simulink model "sinc3_zdomain"  (R2026a)
settings: Solver=FixedStepDiscrete  StopTime=0.5  FixedStep=5e-07
settings Model: Creator=jinwe  LastModifiedBy=jinwe

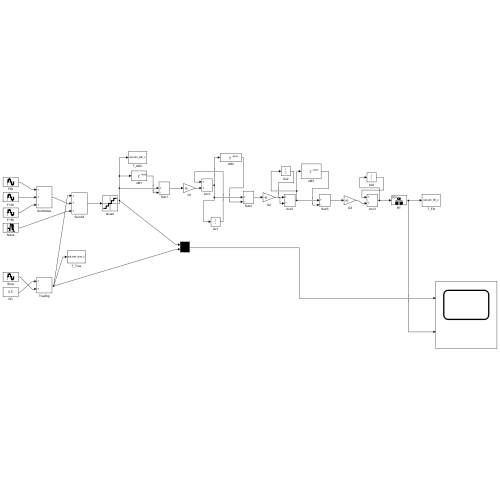
[thumbnail: Simulink's stored preview of the top-level diagram]
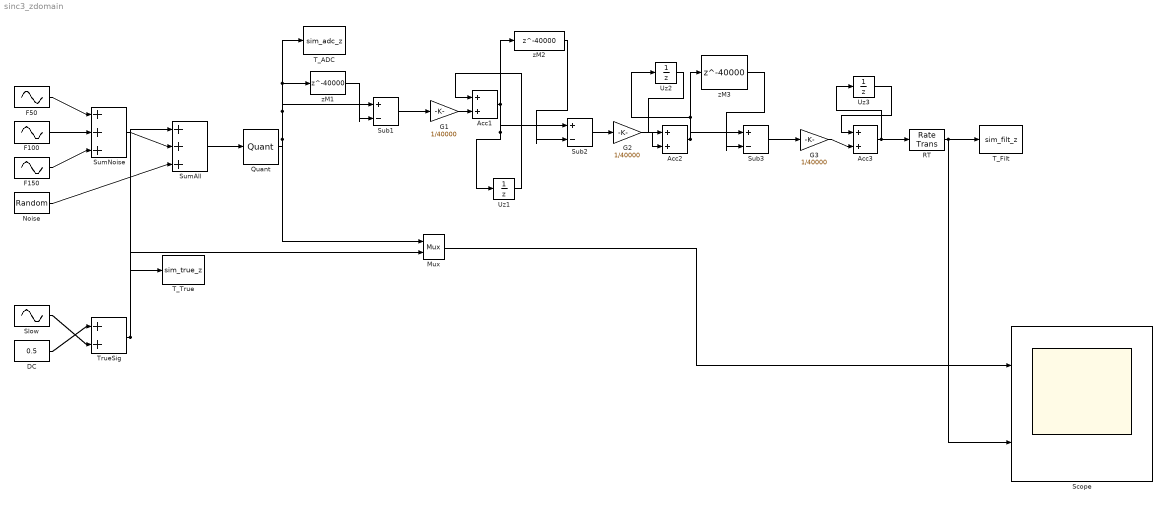
== system sinc3_zdomain ==
  Acc1 : Sum
  Acc2 : Sum
  Acc3 : Sum
  DC : Constant  Value=0.5  SampleTime=5e-07
  F100 : Sin  Amplitude=0.3  Frequency=2*pi*100  SampleTime=5e-07
  F150 : Sin  Amplitude=0.1  Frequency=2*pi*150  SampleTime=5e-07
  F50 : Sin  Amplitude=1.0  Frequency=2*pi*50  SampleTime=5e-07
  G1 : Gain  Gain=1/40000
  G2 : Gain  Gain=1/40000
  G3 : Gain  Gain=1/40000
  Mux : Mux  Inputs=2
  Noise : RandomNumber  Variance=0.0004  SampleTime=5e-07
  Quant : Quantizer  QuantizationInterval=2/2^24
  RT : RateTransition  OutPortSampleTime=0.02
  Scope : Scope  NumInputPorts=2
  Slow : Sin  Amplitude=0.05  Frequency=2*pi*3  SampleTime=5e-07
  Sub1 : Sum  Inputs=|+-
  Sub2 : Sum  Inputs=|+-
  Sub3 : Sum  Inputs=|+-
  SumAll : Sum  Inputs=+++
  SumNoise : Sum  Inputs=+++
  T_ADC : ToWorkspace  VariableName=sim_adc_z  SampleTime=-1
  T_Filt : ToWorkspace  VariableName=sim_filt_z  SampleTime=-1
  T_True : ToWorkspace  VariableName=sim_true_z  SampleTime=-1
  TrueSig : Sum
  Uz1 : UnitDelay  SampleTime=5e-07
  Uz2 : UnitDelay  SampleTime=5e-07
  Uz3 : UnitDelay  SampleTime=5e-07
  zM1 : Delay  DelayLength=40000  SampleTime=5e-07
  zM2 : Delay  DelayLength=40000  SampleTime=5e-07
  zM3 : Delay  DelayLength=40000  SampleTime=5e-07
  wires:
  F50/1 -> SumNoise/1
  F100/1 -> SumNoise/2
  F150/1 -> SumNoise/3
  DC/1 -> TrueSig/1
  Slow/1 -> TrueSig/2
  TrueSig/1 -> SumAll/1, T_True/1, Mux/2
  SumNoise/1 -> SumAll/2
  Noise/1 -> SumAll/3
  SumAll/1 -> Quant/1
  Quant/1 -> zM1/1, T_ADC/1, Sub1/1, Mux/1
  zM1/1 -> Sub1/2
  Sub1/1 -> G1/1
  G1/1 -> Acc1/2
  Acc1/1 -> Uz1/1, Sub2/1, zM2/1
  Uz1/1 -> Acc1/1
  zM2/1 -> Sub2/2
  Sub2/1 -> G2/1
  G2/1 -> Acc2/2
  Acc2/1 -> Uz2/1, zM3/1, Sub3/1
  Uz2/1 -> Acc2/1
  zM3/1 -> Sub3/2
  Sub3/1 -> G3/1
  G3/1 -> Acc3/2
  Acc3/1 -> Uz3/1, RT/1
  Uz3/1 -> Acc3/1
  RT/1 -> T_Filt/1, Scope/2
  Mux/1 -> Scope/1
